simulink model "digiresp_model"  (R2015a)
settings: Solver=ode45  StartTime=0.0  StopTime=20.0  RelTol=1e-3
settings Model: Creator=eechris  LastModifiedBy=ISS-2507830

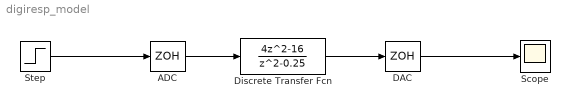
== system digiresp_model ==
  ADC : ZeroOrderHold
  DAC : ZeroOrderHold
  Discrete Transfer Fcn : DiscreteTransferFcn  Numerator="[4, 0,  -16]"  Denominator=[1, 0, -0.25]
  Scope : Scope
  Step : Step  Time=0  SampleTime=0
  wires:
  Discrete Transfer Fcn/1 -> DAC/1
  ADC/1 -> Discrete Transfer Fcn/1
  Step/1 -> ADC/1
  DAC/1 -> Scope/1
